simulink model "dft_8_point"  (R2016b)
settings: Solver=VariableStepDiscrete  StartTime=0.0  StopTime=12/fs  RelTol=1e-3  EnableMultiTasking=on
PreLoadFcn:
  | t = 2;
  | b = 14;
  | 
  | fs = 1;
StartFcn:
  | close all;
StopFcn:
  | % create matrices of Re and Im parts over time - inputs
  | xin_re = [xin_0_re xin_1_re xin_2_re xin_3_re xin_4_re xin_5_re xin_6_re xin_7_re];
  | xin_im = [xin_0_im xin_0_im xin_0_im xin_0_im xin_0_im xin_0_im xin_0_im xin_0_im];
  | 
  | % create matrices of Re and Im parts over time - outputs
  | X_re = [X0_re X1_re X2_re X3_re X4_re X5_re X6_re X7_re];
  | X_im = [X0_im X1_im X2_im X3_im X4_im X5_im X6_im X7_im];
  | 
  | % create vectors of Magnitudes and Angles over time
  | X_mag = [X0_mag X1_mag X2_mag X3_mag X4_mag X5_mag X6_mag X7_mag];
  | X_ang = [X0_ang X1_ang X2_ang X3_ang X4_ang X5_ang X6_ang X7_ang];
  | 
  | 
  | figure(1)
  | hold off
  | plot([0:1:7],xin_re(end,:),'r-o','MarkerFaceColor','r');
  | hold on
  | plot([0:1:7],xin_im(end,:),'b-o','MarkerFaceColor','b');
  | xlabel('Samples');
  | ylabel('Magnitude');
  | title('Input to DFT');
  | legend('Real','Imaginary','Location','EastOutside')
  | grid on;
  | 
  | set(1,'Name','Input to DFT','NumberTitle','off');
  | % setStandardFigSize(1);
  | 
  | figure(2)
  | hold off
  | plot([0:1:7],X_mag(end,:),'k-o','MarkerFaceColor','b');
  | hold on
  | xlabel('Frequency Bin');
  | ylabel('Magnitude');
  | grid on;
  | title('Magnitude DFT Plot');
  | 
  | set(2,'Name','Output of DFT','NumberTitle','off');
  | % setStandardFigSize(2);
libraries: xbsIndex_r4 x955
(part 5 of 8)

== system dft_8_point/cplx mult40 ==
  x : Inport
  AddSub : xbsIndex_r4/AddSub  mode=Addition  use_carryin=off  use_carryout=off  en=off  latency=0  precision=User Defined  arith_type="Signed  (2's comp)"  n_bits=t+b+1  bin_pt=b  quantization=Truncate  overflow=Wrap  use_behavioral_HDL=off  hw_selection=Fabric  pipelined=off  dbl_ovrd=off  block_type=addsub
  AddSub1 : xbsIndex_r4/AddSub  mode=Subtraction  use_carryin=off  use_carryout=off  en=off  latency=0  precision=User Defined  arith_type="Signed  (2's comp)"  n_bits=t+b+1  bin_pt=b  quantization=Truncate  overflow=Wrap  use_behavioral_HDL=off  hw_selection=Fabric  pipelined=off  dbl_ovrd=off  block_type=addsub
  Mult{,1..3} (4 alike) : xbsIndex_r4/Mult  precision=User Defined  arith_type="Signed  (2's comp)"  n_bits=t+b  bin_pt=b  quantization=Truncate  overflow=Wrap  en=off  latency=0  use_behavioral_HDL=off  opt=Speed  use_embedded=on  optimum_pipeline=off  pipeline=on  dbl_ovrd=off  use_rpm=on  placement_style=Triangular  block_type=mult
  Reinterpret : xbsIndex_r4/Reinterpret  force_arith_type=on  arith_type="Signed  (2's comp)"  force_bin_pt=on  bin_pt=b  block_type=reinterpret
      settings: infoedit="Changes signal type without altering the binary representation.   You can changed the signal between signed and unsigned, and relocate the binary point.<br><br>Hardware notes: In hardware this block costs nothing.<br><br>Example:  Suppose the input is 6 bits wide, signed, with 2 fractional bits, and the output is forced to unsigned with 0 fractional bits.  Then an input of -2.0 (1110.00 in binary 2's complement) becomes an output of 56 (111000 in binary)."
  Reinterpret1 : xbsIndex_r4/Reinterpret  force_arith_type=on  arith_type="Signed  (2's comp)"  force_bin_pt=on  bin_pt=b  block_type=reinterpret
      settings: infoedit="Changes signal type without altering the binary representation.   You can changed the signal between signed and unsigned, and relocate the binary point.<br><br>Hardware notes: In hardware this block costs nothing.<br><br>Example:  Suppose the input is 6 bits wide, signed, with 2 fractional bits, and the output is forced to unsigned with 0 fractional bits.  Then an input of -2.0 (1110.00 in binary 2's complement) becomes an output of 56 (111000 in binary)."
  W_imaginary : xbsIndex_r4/Constant  const=imag(Wnk)  gui_display_data_type=Fixed-point  arith_type=Signed (2's comp)  n_bits=t+b  bin_pt=b  preci_type=Single  exp_width=8  frac_width=24  explicit_period=off  period=1  equ=P=C  opselect=C  inp2=PCIN>>17  opr=+  inp1=P  carry=CIN  dbl_ovrd=off  block_type=constant
  W_real : xbsIndex_r4/Constant  const=real(Wnk)  gui_display_data_type=Fixed-point  arith_type=Signed (2's comp)  n_bits=t+b  bin_pt=b  preci_type=Single  exp_width=8  frac_width=24  explicit_period=off  period=1  equ=P=C  opselect=C  inp2=PCIN>>17  opr=+  inp1=P  carry=CIN  dbl_ovrd=off  block_type=constant
  x_imaginary : xbsIndex_r4/Slice  nbits=t+b  boolean_output=off  mode=Lower Bit Location + Width  bit1=0  base1=MSB of Input  bit0=0  base0=LSB of Input  dbl_ovrd=off  block_type=slice
  x_real : xbsIndex_r4/Slice  nbits=t+b  boolean_output=off  mode=Upper Bit Location + Width  bit1=0  base1=MSB of Input  bit0=0  base0=LSB of Input  dbl_ovrd=off  block_type=slice
  xWr : Outport
  xWi : Outport  Port=2
  wires:
  x_real/1 -> Reinterpret/1
  x_imaginary/1 -> Reinterpret1/1
  W_real/1 -> Mult1/2, Mult2/2
  x/1 -> x_real/1, x_imaginary/1
  Reinterpret/1 -> Mult/1, Mult2/1
  Reinterpret1/1 -> Mult1/1, Mult3/1
  W_imaginary/1 -> Mult/2, Mult3/2
  AddSub/1 -> xWi/1
  AddSub1/1 -> xWr/1
  Mult/1 -> AddSub/1
  Mult1/1 -> AddSub/2
  Mult3/1 -> AddSub1/2
  Mult2/1 -> AddSub1/1

== system dft_8_point/cplx mult41 ==
  x : Inport
  AddSub : xbsIndex_r4/AddSub  mode=Addition  use_carryin=off  use_carryout=off  en=off  latency=0  precision=User Defined  arith_type="Signed  (2's comp)"  n_bits=t+b+1  bin_pt=b  quantization=Truncate  overflow=Wrap  use_behavioral_HDL=off  hw_selection=Fabric  pipelined=off  dbl_ovrd=off  block_type=addsub
  AddSub1 : xbsIndex_r4/AddSub  mode=Subtraction  use_carryin=off  use_carryout=off  en=off  latency=0  precision=User Defined  arith_type="Signed  (2's comp)"  n_bits=t+b+1  bin_pt=b  quantization=Truncate  overflow=Wrap  use_behavioral_HDL=off  hw_selection=Fabric  pipelined=off  dbl_ovrd=off  block_type=addsub
  Mult{,1..3} (4 alike) : xbsIndex_r4/Mult  precision=User Defined  arith_type="Signed  (2's comp)"  n_bits=t+b  bin_pt=b  quantization=Truncate  overflow=Wrap  en=off  latency=0  use_behavioral_HDL=off  opt=Speed  use_embedded=on  optimum_pipeline=off  pipeline=on  dbl_ovrd=off  use_rpm=on  placement_style=Triangular  block_type=mult
  Reinterpret : xbsIndex_r4/Reinterpret  force_arith_type=on  arith_type="Signed  (2's comp)"  force_bin_pt=on  bin_pt=b  block_type=reinterpret
      settings: infoedit="Changes signal type without altering the binary representation.   You can changed the signal between signed and unsigned, and relocate the binary point.<br><br>Hardware notes: In hardware this block costs nothing.<br><br>Example:  Suppose the input is 6 bits wide, signed, with 2 fractional bits, and the output is forced to unsigned with 0 fractional bits.  Then an input of -2.0 (1110.00 in binary 2's complement) becomes an output of 56 (111000 in binary)."
  Reinterpret1 : xbsIndex_r4/Reinterpret  force_arith_type=on  arith_type="Signed  (2's comp)"  force_bin_pt=on  bin_pt=b  block_type=reinterpret
      settings: infoedit="Changes signal type without altering the binary representation.   You can changed the signal between signed and unsigned, and relocate the binary point.<br><br>Hardware notes: In hardware this block costs nothing.<br><br>Example:  Suppose the input is 6 bits wide, signed, with 2 fractional bits, and the output is forced to unsigned with 0 fractional bits.  Then an input of -2.0 (1110.00 in binary 2's complement) becomes an output of 56 (111000 in binary)."
  W_imaginary : xbsIndex_r4/Constant  const=imag(Wnk)  gui_display_data_type=Fixed-point  arith_type=Signed (2's comp)  n_bits=t+b  bin_pt=b  preci_type=Single  exp_width=8  frac_width=24  explicit_period=off  period=1  equ=P=C  opselect=C  inp2=PCIN>>17  opr=+  inp1=P  carry=CIN  dbl_ovrd=off  block_type=constant
  W_real : xbsIndex_r4/Constant  const=real(Wnk)  gui_display_data_type=Fixed-point  arith_type=Signed (2's comp)  n_bits=t+b  bin_pt=b  preci_type=Single  exp_width=8  frac_width=24  explicit_period=off  period=1  equ=P=C  opselect=C  inp2=PCIN>>17  opr=+  inp1=P  carry=CIN  dbl_ovrd=off  block_type=constant
  x_imaginary : xbsIndex_r4/Slice  nbits=t+b  boolean_output=off  mode=Lower Bit Location + Width  bit1=0  base1=MSB of Input  bit0=0  base0=LSB of Input  dbl_ovrd=off  block_type=slice
  x_real : xbsIndex_r4/Slice  nbits=t+b  boolean_output=off  mode=Upper Bit Location + Width  bit1=0  base1=MSB of Input  bit0=0  base0=LSB of Input  dbl_ovrd=off  block_type=slice
  xWr : Outport
  xWi : Outport  Port=2
  wires:
  x_real/1 -> Reinterpret/1
  x_imaginary/1 -> Reinterpret1/1
  W_real/1 -> Mult1/2, Mult2/2
  x/1 -> x_real/1, x_imaginary/1
  Reinterpret/1 -> Mult/1, Mult2/1
  Reinterpret1/1 -> Mult1/1, Mult3/1
  W_imaginary/1 -> Mult/2, Mult3/2
  AddSub/1 -> xWi/1
  AddSub1/1 -> xWr/1
  Mult/1 -> AddSub/1
  Mult1/1 -> AddSub/2
  Mult3/1 -> AddSub1/2
  Mult2/1 -> AddSub1/1

== system dft_8_point/cplx mult42 ==
  x : Inport
  AddSub : xbsIndex_r4/AddSub  mode=Addition  use_carryin=off  use_carryout=off  en=off  latency=0  precision=User Defined  arith_type="Signed  (2's comp)"  n_bits=t+b+1  bin_pt=b  quantization=Truncate  overflow=Wrap  use_behavioral_HDL=off  hw_selection=Fabric  pipelined=off  dbl_ovrd=off  block_type=addsub
  AddSub1 : xbsIndex_r4/AddSub  mode=Subtraction  use_carryin=off  use_carryout=off  en=off  latency=0  precision=User Defined  arith_type="Signed  (2's comp)"  n_bits=t+b+1  bin_pt=b  quantization=Truncate  overflow=Wrap  use_behavioral_HDL=off  hw_selection=Fabric  pipelined=off  dbl_ovrd=off  block_type=addsub
  Mult{,1..3} (4 alike) : xbsIndex_r4/Mult  precision=User Defined  arith_type="Signed  (2's comp)"  n_bits=t+b  bin_pt=b  quantization=Truncate  overflow=Wrap  en=off  latency=0  use_behavioral_HDL=off  opt=Speed  use_embedded=on  optimum_pipeline=off  pipeline=on  dbl_ovrd=off  use_rpm=on  placement_style=Triangular  block_type=mult
  Reinterpret : xbsIndex_r4/Reinterpret  force_arith_type=on  arith_type="Signed  (2's comp)"  force_bin_pt=on  bin_pt=b  block_type=reinterpret
      settings: infoedit="Changes signal type without altering the binary representation.   You can changed the signal between signed and unsigned, and relocate the binary point.<br><br>Hardware notes: In hardware this block costs nothing.<br><br>Example:  Suppose the input is 6 bits wide, signed, with 2 fractional bits, and the output is forced to unsigned with 0 fractional bits.  Then an input of -2.0 (1110.00 in binary 2's complement) becomes an output of 56 (111000 in binary)."
  Reinterpret1 : xbsIndex_r4/Reinterpret  force_arith_type=on  arith_type="Signed  (2's comp)"  force_bin_pt=on  bin_pt=b  block_type=reinterpret
      settings: infoedit="Changes signal type without altering the binary representation.   You can changed the signal between signed and unsigned, and relocate the binary point.<br><br>Hardware notes: In hardware this block costs nothing.<br><br>Example:  Suppose the input is 6 bits wide, signed, with 2 fractional bits, and the output is forced to unsigned with 0 fractional bits.  Then an input of -2.0 (1110.00 in binary 2's complement) becomes an output of 56 (111000 in binary)."
  W_imaginary : xbsIndex_r4/Constant  const=imag(Wnk)  gui_display_data_type=Fixed-point  arith_type=Signed (2's comp)  n_bits=t+b  bin_pt=b  preci_type=Single  exp_width=8  frac_width=24  explicit_period=off  period=1  equ=P=C  opselect=C  inp2=PCIN>>17  opr=+  inp1=P  carry=CIN  dbl_ovrd=off  block_type=constant
  W_real : xbsIndex_r4/Constant  const=real(Wnk)  gui_display_data_type=Fixed-point  arith_type=Signed (2's comp)  n_bits=t+b  bin_pt=b  preci_type=Single  exp_width=8  frac_width=24  explicit_period=off  period=1  equ=P=C  opselect=C  inp2=PCIN>>17  opr=+  inp1=P  carry=CIN  dbl_ovrd=off  block_type=constant
  x_imaginary : xbsIndex_r4/Slice  nbits=t+b  boolean_output=off  mode=Lower Bit Location + Width  bit1=0  base1=MSB of Input  bit0=0  base0=LSB of Input  dbl_ovrd=off  block_type=slice
  x_real : xbsIndex_r4/Slice  nbits=t+b  boolean_output=off  mode=Upper Bit Location + Width  bit1=0  base1=MSB of Input  bit0=0  base0=LSB of Input  dbl_ovrd=off  block_type=slice
  xWr : Outport
  xWi : Outport  Port=2
  wires:
  x_real/1 -> Reinterpret/1
  x_imaginary/1 -> Reinterpret1/1
  W_real/1 -> Mult1/2, Mult2/2
  x/1 -> x_real/1, x_imaginary/1
  Reinterpret/1 -> Mult/1, Mult2/1
  Reinterpret1/1 -> Mult1/1, Mult3/1
  W_imaginary/1 -> Mult/2, Mult3/2
  AddSub/1 -> xWi/1
  AddSub1/1 -> xWr/1
  Mult/1 -> AddSub/1
  Mult1/1 -> AddSub/2
  Mult3/1 -> AddSub1/2
  Mult2/1 -> AddSub1/1

== system dft_8_point/cplx mult43 ==
  x : Inport
  AddSub : xbsIndex_r4/AddSub  mode=Addition  use_carryin=off  use_carryout=off  en=off  latency=0  precision=User Defined  arith_type="Signed  (2's comp)"  n_bits=t+b+1  bin_pt=b  quantization=Truncate  overflow=Wrap  use_behavioral_HDL=off  hw_selection=Fabric  pipelined=off  dbl_ovrd=off  block_type=addsub
  AddSub1 : xbsIndex_r4/AddSub  mode=Subtraction  use_carryin=off  use_carryout=off  en=off  latency=0  precision=User Defined  arith_type="Signed  (2's comp)"  n_bits=t+b+1  bin_pt=b  quantization=Truncate  overflow=Wrap  use_behavioral_HDL=off  hw_selection=Fabric  pipelined=off  dbl_ovrd=off  block_type=addsub
  Mult{,1..3} (4 alike) : xbsIndex_r4/Mult  precision=User Defined  arith_type="Signed  (2's comp)"  n_bits=t+b  bin_pt=b  quantization=Truncate  overflow=Wrap  en=off  latency=0  use_behavioral_HDL=off  opt=Speed  use_embedded=on  optimum_pipeline=off  pipeline=on  dbl_ovrd=off  use_rpm=on  placement_style=Triangular  block_type=mult
  Reinterpret : xbsIndex_r4/Reinterpret  force_arith_type=on  arith_type="Signed  (2's comp)"  force_bin_pt=on  bin_pt=b  block_type=reinterpret
      settings: infoedit="Changes signal type without altering the binary representation.   You can changed the signal between signed and unsigned, and relocate the binary point.<br><br>Hardware notes: In hardware this block costs nothing.<br><br>Example:  Suppose the input is 6 bits wide, signed, with 2 fractional bits, and the output is forced to unsigned with 0 fractional bits.  Then an input of -2.0 (1110.00 in binary 2's complement) becomes an output of 56 (111000 in binary)."
  Reinterpret1 : xbsIndex_r4/Reinterpret  force_arith_type=on  arith_type="Signed  (2's comp)"  force_bin_pt=on  bin_pt=b  block_type=reinterpret
      settings: infoedit="Changes signal type without altering the binary representation.   You can changed the signal between signed and unsigned, and relocate the binary point.<br><br>Hardware notes: In hardware this block costs nothing.<br><br>Example:  Suppose the input is 6 bits wide, signed, with 2 fractional bits, and the output is forced to unsigned with 0 fractional bits.  Then an input of -2.0 (1110.00 in binary 2's complement) becomes an output of 56 (111000 in binary)."
  W_imaginary : xbsIndex_r4/Constant  const=imag(Wnk)  gui_display_data_type=Fixed-point  arith_type=Signed (2's comp)  n_bits=t+b  bin_pt=b  preci_type=Single  exp_width=8  frac_width=24  explicit_period=off  period=1  equ=P=C  opselect=C  inp2=PCIN>>17  opr=+  inp1=P  carry=CIN  dbl_ovrd=off  block_type=constant
  W_real : xbsIndex_r4/Constant  const=real(Wnk)  gui_display_data_type=Fixed-point  arith_type=Signed (2's comp)  n_bits=t+b  bin_pt=b  preci_type=Single  exp_width=8  frac_width=24  explicit_period=off  period=1  equ=P=C  opselect=C  inp2=PCIN>>17  opr=+  inp1=P  carry=CIN  dbl_ovrd=off  block_type=constant
  x_imaginary : xbsIndex_r4/Slice  nbits=t+b  boolean_output=off  mode=Lower Bit Location + Width  bit1=0  base1=MSB of Input  bit0=0  base0=LSB of Input  dbl_ovrd=off  block_type=slice
  x_real : xbsIndex_r4/Slice  nbits=t+b  boolean_output=off  mode=Upper Bit Location + Width  bit1=0  base1=MSB of Input  bit0=0  base0=LSB of Input  dbl_ovrd=off  block_type=slice
  xWr : Outport
  xWi : Outport  Port=2
  wires:
  x_real/1 -> Reinterpret/1
  x_imaginary/1 -> Reinterpret1/1
  W_real/1 -> Mult1/2, Mult2/2
  x/1 -> x_real/1, x_imaginary/1
  Reinterpret/1 -> Mult/1, Mult2/1
  Reinterpret1/1 -> Mult1/1, Mult3/1
  W_imaginary/1 -> Mult/2, Mult3/2
  AddSub/1 -> xWi/1
  AddSub1/1 -> xWr/1
  Mult/1 -> AddSub/1
  Mult1/1 -> AddSub/2
  Mult3/1 -> AddSub1/2
  Mult2/1 -> AddSub1/1

== system dft_8_point/cplx mult44 ==
  x : Inport
  AddSub : xbsIndex_r4/AddSub  mode=Addition  use_carryin=off  use_carryout=off  en=off  latency=0  precision=User Defined  arith_type="Signed  (2's comp)"  n_bits=t+b+1  bin_pt=b  quantization=Truncate  overflow=Wrap  use_behavioral_HDL=off  hw_selection=Fabric  pipelined=off  dbl_ovrd=off  block_type=addsub
  AddSub1 : xbsIndex_r4/AddSub  mode=Subtraction  use_carryin=off  use_carryout=off  en=off  latency=0  precision=User Defined  arith_type="Signed  (2's comp)"  n_bits=t+b+1  bin_pt=b  quantization=Truncate  overflow=Wrap  use_behavioral_HDL=off  hw_selection=Fabric  pipelined=off  dbl_ovrd=off  block_type=addsub
  Mult{,1..3} (4 alike) : xbsIndex_r4/Mult  precision=User Defined  arith_type="Signed  (2's comp)"  n_bits=t+b  bin_pt=b  quantization=Truncate  overflow=Wrap  en=off  latency=0  use_behavioral_HDL=off  opt=Speed  use_embedded=on  optimum_pipeline=off  pipeline=on  dbl_ovrd=off  use_rpm=on  placement_style=Triangular  block_type=mult
  Reinterpret : xbsIndex_r4/Reinterpret  force_arith_type=on  arith_type="Signed  (2's comp)"  force_bin_pt=on  bin_pt=b  block_type=reinterpret
      settings: infoedit="Changes signal type without altering the binary representation.   You can changed the signal between signed and unsigned, and relocate the binary point.<br><br>Hardware notes: In hardware this block costs nothing.<br><br>Example:  Suppose the input is 6 bits wide, signed, with 2 fractional bits, and the output is forced to unsigned with 0 fractional bits.  Then an input of -2.0 (1110.00 in binary 2's complement) becomes an output of 56 (111000 in binary)."
  Reinterpret1 : xbsIndex_r4/Reinterpret  force_arith_type=on  arith_type="Signed  (2's comp)"  force_bin_pt=on  bin_pt=b  block_type=reinterpret
      settings: infoedit="Changes signal type without altering the binary representation.   You can changed the signal between signed and unsigned, and relocate the binary point.<br><br>Hardware notes: In hardware this block costs nothing.<br><br>Example:  Suppose the input is 6 bits wide, signed, with 2 fractional bits, and the output is forced to unsigned with 0 fractional bits.  Then an input of -2.0 (1110.00 in binary 2's complement) becomes an output of 56 (111000 in binary)."
  W_imaginary : xbsIndex_r4/Constant  const=imag(Wnk)  gui_display_data_type=Fixed-point  arith_type=Signed (2's comp)  n_bits=t+b  bin_pt=b  preci_type=Single  exp_width=8  frac_width=24  explicit_period=off  period=1  equ=P=C  opselect=C  inp2=PCIN>>17  opr=+  inp1=P  carry=CIN  dbl_ovrd=off  block_type=constant
  W_real : xbsIndex_r4/Constant  const=real(Wnk)  gui_display_data_type=Fixed-point  arith_type=Signed (2's comp)  n_bits=t+b  bin_pt=b  preci_type=Single  exp_width=8  frac_width=24  explicit_period=off  period=1  equ=P=C  opselect=C  inp2=PCIN>>17  opr=+  inp1=P  carry=CIN  dbl_ovrd=off  block_type=constant
  x_imaginary : xbsIndex_r4/Slice  nbits=t+b  boolean_output=off  mode=Lower Bit Location + Width  bit1=0  base1=MSB of Input  bit0=0  base0=LSB of Input  dbl_ovrd=off  block_type=slice
  x_real : xbsIndex_r4/Slice  nbits=t+b  boolean_output=off  mode=Upper Bit Location + Width  bit1=0  base1=MSB of Input  bit0=0  base0=LSB of Input  dbl_ovrd=off  block_type=slice
  xWr : Outport
  xWi : Outport  Port=2
  wires:
  x_real/1 -> Reinterpret/1
  x_imaginary/1 -> Reinterpret1/1
  W_real/1 -> Mult1/2, Mult2/2
  x/1 -> x_real/1, x_imaginary/1
  Reinterpret/1 -> Mult/1, Mult2/1
  Reinterpret1/1 -> Mult1/1, Mult3/1
  W_imaginary/1 -> Mult/2, Mult3/2
  AddSub/1 -> xWi/1
  AddSub1/1 -> xWr/1
  Mult/1 -> AddSub/1
  Mult1/1 -> AddSub/2
  Mult3/1 -> AddSub1/2
  Mult2/1 -> AddSub1/1

== system dft_8_point/cplx mult45 ==
  x : Inport
  AddSub : xbsIndex_r4/AddSub  mode=Addition  use_carryin=off  use_carryout=off  en=off  latency=0  precision=User Defined  arith_type="Signed  (2's comp)"  n_bits=t+b+1  bin_pt=b  quantization=Truncate  overflow=Wrap  use_behavioral_HDL=off  hw_selection=Fabric  pipelined=off  dbl_ovrd=off  block_type=addsub
  AddSub1 : xbsIndex_r4/AddSub  mode=Subtraction  use_carryin=off  use_carryout=off  en=off  latency=0  precision=User Defined  arith_type="Signed  (2's comp)"  n_bits=t+b+1  bin_pt=b  quantization=Truncate  overflow=Wrap  use_behavioral_HDL=off  hw_selection=Fabric  pipelined=off  dbl_ovrd=off  block_type=addsub
  Mult{,1..3} (4 alike) : xbsIndex_r4/Mult  precision=User Defined  arith_type="Signed  (2's comp)"  n_bits=t+b  bin_pt=b  quantization=Truncate  overflow=Wrap  en=off  latency=0  use_behavioral_HDL=off  opt=Speed  use_embedded=on  optimum_pipeline=off  pipeline=on  dbl_ovrd=off  use_rpm=on  placement_style=Triangular  block_type=mult
  Reinterpret : xbsIndex_r4/Reinterpret  force_arith_type=on  arith_type="Signed  (2's comp)"  force_bin_pt=on  bin_pt=b  block_type=reinterpret
      settings: infoedit="Changes signal type without altering the binary representation.   You can changed the signal between signed and unsigned, and relocate the binary point.<br><br>Hardware notes: In hardware this block costs nothing.<br><br>Example:  Suppose the input is 6 bits wide, signed, with 2 fractional bits, and the output is forced to unsigned with 0 fractional bits.  Then an input of -2.0 (1110.00 in binary 2's complement) becomes an output of 56 (111000 in binary)."
  Reinterpret1 : xbsIndex_r4/Reinterpret  force_arith_type=on  arith_type="Signed  (2's comp)"  force_bin_pt=on  bin_pt=b  block_type=reinterpret
      settings: infoedit="Changes signal type without altering the binary representation.   You can changed the signal between signed and unsigned, and relocate the binary point.<br><br>Hardware notes: In hardware this block costs nothing.<br><br>Example:  Suppose the input is 6 bits wide, signed, with 2 fractional bits, and the output is forced to unsigned with 0 fractional bits.  Then an input of -2.0 (1110.00 in binary 2's complement) becomes an output of 56 (111000 in binary)."
  W_imaginary : xbsIndex_r4/Constant  const=imag(Wnk)  gui_display_data_type=Fixed-point  arith_type=Signed (2's comp)  n_bits=t+b  bin_pt=b  preci_type=Single  exp_width=8  frac_width=24  explicit_period=off  period=1  equ=P=C  opselect=C  inp2=PCIN>>17  opr=+  inp1=P  carry=CIN  dbl_ovrd=off  block_type=constant
  W_real : xbsIndex_r4/Constant  const=real(Wnk)  gui_display_data_type=Fixed-point  arith_type=Signed (2's comp)  n_bits=t+b  bin_pt=b  preci_type=Single  exp_width=8  frac_width=24  explicit_period=off  period=1  equ=P=C  opselect=C  inp2=PCIN>>17  opr=+  inp1=P  carry=CIN  dbl_ovrd=off  block_type=constant
  x_imaginary : xbsIndex_r4/Slice  nbits=t+b  boolean_output=off  mode=Lower Bit Location + Width  bit1=0  base1=MSB of Input  bit0=0  base0=LSB of Input  dbl_ovrd=off  block_type=slice
  x_real : xbsIndex_r4/Slice  nbits=t+b  boolean_output=off  mode=Upper Bit Location + Width  bit1=0  base1=MSB of Input  bit0=0  base0=LSB of Input  dbl_ovrd=off  block_type=slice
  xWr : Outport
  xWi : Outport  Port=2
  wires:
  x_real/1 -> Reinterpret/1
  x_imaginary/1 -> Reinterpret1/1
  W_real/1 -> Mult1/2, Mult2/2
  x/1 -> x_real/1, x_imaginary/1
  Reinterpret/1 -> Mult/1, Mult2/1
  Reinterpret1/1 -> Mult1/1, Mult3/1
  W_imaginary/1 -> Mult/2, Mult3/2
  AddSub/1 -> xWi/1
  AddSub1/1 -> xWr/1
  Mult/1 -> AddSub/1
  Mult1/1 -> AddSub/2
  Mult3/1 -> AddSub1/2
  Mult2/1 -> AddSub1/1

== system dft_8_point/cplx mult46 ==
  x : Inport
  AddSub : xbsIndex_r4/AddSub  mode=Addition  use_carryin=off  use_carryout=off  en=off  latency=0  precision=User Defined  arith_type="Signed  (2's comp)"  n_bits=t+b+1  bin_pt=b  quantization=Truncate  overflow=Wrap  use_behavioral_HDL=off  hw_selection=Fabric  pipelined=off  dbl_ovrd=off  block_type=addsub
  AddSub1 : xbsIndex_r4/AddSub  mode=Subtraction  use_carryin=off  use_carryout=off  en=off  latency=0  precision=User Defined  arith_type="Signed  (2's comp)"  n_bits=t+b+1  bin_pt=b  quantization=Truncate  overflow=Wrap  use_behavioral_HDL=off  hw_selection=Fabric  pipelined=off  dbl_ovrd=off  block_type=addsub
  Mult{,1..3} (4 alike) : xbsIndex_r4/Mult  precision=User Defined  arith_type="Signed  (2's comp)"  n_bits=t+b  bin_pt=b  quantization=Truncate  overflow=Wrap  en=off  latency=0  use_behavioral_HDL=off  opt=Speed  use_embedded=on  optimum_pipeline=off  pipeline=on  dbl_ovrd=off  use_rpm=on  placement_style=Triangular  block_type=mult
  Reinterpret : xbsIndex_r4/Reinterpret  force_arith_type=on  arith_type="Signed  (2's comp)"  force_bin_pt=on  bin_pt=b  block_type=reinterpret
      settings: infoedit="Changes signal type without altering the binary representation.   You can changed the signal between signed and unsigned, and relocate the binary point.<br><br>Hardware notes: In hardware this block costs nothing.<br><br>Example:  Suppose the input is 6 bits wide, signed, with 2 fractional bits, and the output is forced to unsigned with 0 fractional bits.  Then an input of -2.0 (1110.00 in binary 2's complement) becomes an output of 56 (111000 in binary)."
  Reinterpret1 : xbsIndex_r4/Reinterpret  force_arith_type=on  arith_type="Signed  (2's comp)"  force_bin_pt=on  bin_pt=b  block_type=reinterpret
      settings: infoedit="Changes signal type without altering the binary representation.   You can changed the signal between signed and unsigned, and relocate the binary point.<br><br>Hardware notes: In hardware this block costs nothing.<br><br>Example:  Suppose the input is 6 bits wide, signed, with 2 fractional bits, and the output is forced to unsigned with 0 fractional bits.  Then an input of -2.0 (1110.00 in binary 2's complement) becomes an output of 56 (111000 in binary)."
  W_imaginary : xbsIndex_r4/Constant  const=imag(Wnk)  gui_display_data_type=Fixed-point  arith_type=Signed (2's comp)  n_bits=t+b  bin_pt=b  preci_type=Single  exp_width=8  frac_width=24  explicit_period=off  period=1  equ=P=C  opselect=C  inp2=PCIN>>17  opr=+  inp1=P  carry=CIN  dbl_ovrd=off  block_type=constant
  W_real : xbsIndex_r4/Constant  const=real(Wnk)  gui_display_data_type=Fixed-point  arith_type=Signed (2's comp)  n_bits=t+b  bin_pt=b  preci_type=Single  exp_width=8  frac_width=24  explicit_period=off  period=1  equ=P=C  opselect=C  inp2=PCIN>>17  opr=+  inp1=P  carry=CIN  dbl_ovrd=off  block_type=constant
  x_imaginary : xbsIndex_r4/Slice  nbits=t+b  boolean_output=off  mode=Lower Bit Location + Width  bit1=0  base1=MSB of Input  bit0=0  base0=LSB of Input  dbl_ovrd=off  block_type=slice
  x_real : xbsIndex_r4/Slice  nbits=t+b  boolean_output=off  mode=Upper Bit Location + Width  bit1=0  base1=MSB of Input  bit0=0  base0=LSB of Input  dbl_ovrd=off  block_type=slice
  xWr : Outport
  xWi : Outport  Port=2
  wires:
  x_real/1 -> Reinterpret/1
  x_imaginary/1 -> Reinterpret1/1
  W_real/1 -> Mult1/2, Mult2/2
  x/1 -> x_real/1, x_imaginary/1
  Reinterpret/1 -> Mult/1, Mult2/1
  Reinterpret1/1 -> Mult1/1, Mult3/1
  W_imaginary/1 -> Mult/2, Mult3/2
  AddSub/1 -> xWi/1
  AddSub1/1 -> xWr/1
  Mult/1 -> AddSub/1
  Mult1/1 -> AddSub/2
  Mult3/1 -> AddSub1/2
  Mult2/1 -> AddSub1/1

== system dft_8_point/cplx mult47 ==
  x : Inport
  AddSub : xbsIndex_r4/AddSub  mode=Addition  use_carryin=off  use_carryout=off  en=off  latency=0  precision=User Defined  arith_type="Signed  (2's comp)"  n_bits=t+b+1  bin_pt=b  quantization=Truncate  overflow=Wrap  use_behavioral_HDL=off  hw_selection=Fabric  pipelined=off  dbl_ovrd=off  block_type=addsub
  AddSub1 : xbsIndex_r4/AddSub  mode=Subtraction  use_carryin=off  use_carryout=off  en=off  latency=0  precision=User Defined  arith_type="Signed  (2's comp)"  n_bits=t+b+1  bin_pt=b  quantization=Truncate  overflow=Wrap  use_behavioral_HDL=off  hw_selection=Fabric  pipelined=off  dbl_ovrd=off  block_type=addsub
  Mult{,1..3} (4 alike) : xbsIndex_r4/Mult  precision=User Defined  arith_type="Signed  (2's comp)"  n_bits=t+b  bin_pt=b  quantization=Truncate  overflow=Wrap  en=off  latency=0  use_behavioral_HDL=off  opt=Speed  use_embedded=on  optimum_pipeline=off  pipeline=on  dbl_ovrd=off  use_rpm=on  placement_style=Triangular  block_type=mult
  Reinterpret : xbsIndex_r4/Reinterpret  force_arith_type=on  arith_type="Signed  (2's comp)"  force_bin_pt=on  bin_pt=b  block_type=reinterpret
      settings: infoedit="Changes signal type without altering the binary representation.   You can changed the signal between signed and unsigned, and relocate the binary point.<br><br>Hardware notes: In hardware this block costs nothing.<br><br>Example:  Suppose the input is 6 bits wide, signed, with 2 fractional bits, and the output is forced to unsigned with 0 fractional bits.  Then an input of -2.0 (1110.00 in binary 2's complement) becomes an output of 56 (111000 in binary)."
  Reinterpret1 : xbsIndex_r4/Reinterpret  force_arith_type=on  arith_type="Signed  (2's comp)"  force_bin_pt=on  bin_pt=b  block_type=reinterpret
      settings: infoedit="Changes signal type without altering the binary representation.   You can changed the signal between signed and unsigned, and relocate the binary point.<br><br>Hardware notes: In hardware this block costs nothing.<br><br>Example:  Suppose the input is 6 bits wide, signed, with 2 fractional bits, and the output is forced to unsigned with 0 fractional bits.  Then an input of -2.0 (1110.00 in binary 2's complement) becomes an output of 56 (111000 in binary)."
  W_imaginary : xbsIndex_r4/Constant  const=imag(Wnk)  gui_display_data_type=Fixed-point  arith_type=Signed (2's comp)  n_bits=t+b  bin_pt=b  preci_type=Single  exp_width=8  frac_width=24  explicit_period=off  period=1  equ=P=C  opselect=C  inp2=PCIN>>17  opr=+  inp1=P  carry=CIN  dbl_ovrd=off  block_type=constant
  W_real : xbsIndex_r4/Constant  const=real(Wnk)  gui_display_data_type=Fixed-point  arith_type=Signed (2's comp)  n_bits=t+b  bin_pt=b  preci_type=Single  exp_width=8  frac_width=24  explicit_period=off  period=1  equ=P=C  opselect=C  inp2=PCIN>>17  opr=+  inp1=P  carry=CIN  dbl_ovrd=off  block_type=constant
  x_imaginary : xbsIndex_r4/Slice  nbits=t+b  boolean_output=off  mode=Lower Bit Location + Width  bit1=0  base1=MSB of Input  bit0=0  base0=LSB of Input  dbl_ovrd=off  block_type=slice
  x_real : xbsIndex_r4/Slice  nbits=t+b  boolean_output=off  mode=Upper Bit Location + Width  bit1=0  base1=MSB of Input  bit0=0  base0=LSB of Input  dbl_ovrd=off  block_type=slice
  xWr : Outport
  xWi : Outport  Port=2
  wires:
  x_real/1 -> Reinterpret/1
  x_imaginary/1 -> Reinterpret1/1
  W_real/1 -> Mult1/2, Mult2/2
  x/1 -> x_real/1, x_imaginary/1
  Reinterpret/1 -> Mult/1, Mult2/1
  Reinterpret1/1 -> Mult1/1, Mult3/1
  W_imaginary/1 -> Mult/2, Mult3/2
  AddSub/1 -> xWi/1
  AddSub1/1 -> xWr/1
  Mult/1 -> AddSub/1
  Mult1/1 -> AddSub/2
  Mult3/1 -> AddSub1/2
  Mult2/1 -> AddSub1/1

== system dft_8_point/cplx mult48 ==
  x : Inport
  AddSub : xbsIndex_r4/AddSub  mode=Addition  use_carryin=off  use_carryout=off  en=off  latency=0  precision=User Defined  arith_type="Signed  (2's comp)"  n_bits=t+b+1  bin_pt=b  quantization=Truncate  overflow=Wrap  use_behavioral_HDL=off  hw_selection=Fabric  pipelined=off  dbl_ovrd=off  block_type=addsub
  AddSub1 : xbsIndex_r4/AddSub  mode=Subtraction  use_carryin=off  use_carryout=off  en=off  latency=0  precision=User Defined  arith_type="Signed  (2's comp)"  n_bits=t+b+1  bin_pt=b  quantization=Truncate  overflow=Wrap  use_behavioral_HDL=off  hw_selection=Fabric  pipelined=off  dbl_ovrd=off  block_type=addsub
  Mult{,1..3} (4 alike) : xbsIndex_r4/Mult  precision=User Defined  arith_type="Signed  (2's comp)"  n_bits=t+b  bin_pt=b  quantization=Truncate  overflow=Wrap  en=off  latency=0  use_behavioral_HDL=off  opt=Speed  use_embedded=on  optimum_pipeline=off  pipeline=on  dbl_ovrd=off  use_rpm=on  placement_style=Triangular  block_type=mult
  Reinterpret : xbsIndex_r4/Reinterpret  force_arith_type=on  arith_type="Signed  (2's comp)"  force_bin_pt=on  bin_pt=b  block_type=reinterpret
      settings: infoedit="Changes signal type without altering the binary representation.   You can changed the signal between signed and unsigned, and relocate the binary point.<br><br>Hardware notes: In hardware this block costs nothing.<br><br>Example:  Suppose the input is 6 bits wide, signed, with 2 fractional bits, and the output is forced to unsigned with 0 fractional bits.  Then an input of -2.0 (1110.00 in binary 2's complement) becomes an output of 56 (111000 in binary)."
  Reinterpret1 : xbsIndex_r4/Reinterpret  force_arith_type=on  arith_type="Signed  (2's comp)"  force_bin_pt=on  bin_pt=b  block_type=reinterpret
      settings: infoedit="Changes signal type without altering the binary representation.   You can changed the signal between signed and unsigned, and relocate the binary point.<br><br>Hardware notes: In hardware this block costs nothing.<br><br>Example:  Suppose the input is 6 bits wide, signed, with 2 fractional bits, and the output is forced to unsigned with 0 fractional bits.  Then an input of -2.0 (1110.00 in binary 2's complement) becomes an output of 56 (111000 in binary)."
  W_imaginary : xbsIndex_r4/Constant  const=imag(Wnk)  gui_display_data_type=Fixed-point  arith_type=Signed (2's comp)  n_bits=t+b  bin_pt=b  preci_type=Single  exp_width=8  frac_width=24  explicit_period=off  period=1  equ=P=C  opselect=C  inp2=PCIN>>17  opr=+  inp1=P  carry=CIN  dbl_ovrd=off  block_type=constant
  W_real : xbsIndex_r4/Constant  const=real(Wnk)  gui_display_data_type=Fixed-point  arith_type=Signed (2's comp)  n_bits=t+b  bin_pt=b  preci_type=Single  exp_width=8  frac_width=24  explicit_period=off  period=1  equ=P=C  opselect=C  inp2=PCIN>>17  opr=+  inp1=P  carry=CIN  dbl_ovrd=off  block_type=constant
  x_imaginary : xbsIndex_r4/Slice  nbits=t+b  boolean_output=off  mode=Lower Bit Location + Width  bit1=0  base1=MSB of Input  bit0=0  base0=LSB of Input  dbl_ovrd=off  block_type=slice
  x_real : xbsIndex_r4/Slice  nbits=t+b  boolean_output=off  mode=Upper Bit Location + Width  bit1=0  base1=MSB of Input  bit0=0  base0=LSB of Input  dbl_ovrd=off  block_type=slice
  xWr : Outport
  xWi : Outport  Port=2
  wires:
  x_real/1 -> Reinterpret/1
  x_imaginary/1 -> Reinterpret1/1
  W_real/1 -> Mult1/2, Mult2/2
  x/1 -> x_real/1, x_imaginary/1
  Reinterpret/1 -> Mult/1, Mult2/1
  Reinterpret1/1 -> Mult1/1, Mult3/1
  W_imaginary/1 -> Mult/2, Mult3/2
  AddSub/1 -> xWi/1
  AddSub1/1 -> xWr/1
  Mult/1 -> AddSub/1
  Mult1/1 -> AddSub/2
  Mult3/1 -> AddSub1/2
  Mult2/1 -> AddSub1/1

== system dft_8_point/cplx mult49 ==
  x : Inport
  AddSub : xbsIndex_r4/AddSub  mode=Addition  use_carryin=off  use_carryout=off  en=off  latency=0  precision=User Defined  arith_type="Signed  (2's comp)"  n_bits=t+b+1  bin_pt=b  quantization=Truncate  overflow=Wrap  use_behavioral_HDL=off  hw_selection=Fabric  pipelined=off  dbl_ovrd=off  block_type=addsub
  AddSub1 : xbsIndex_r4/AddSub  mode=Subtraction  use_carryin=off  use_carryout=off  en=off  latency=0  precision=User Defined  arith_type="Signed  (2's comp)"  n_bits=t+b+1  bin_pt=b  quantization=Truncate  overflow=Wrap  use_behavioral_HDL=off  hw_selection=Fabric  pipelined=off  dbl_ovrd=off  block_type=addsub
  Mult{,1..3} (4 alike) : xbsIndex_r4/Mult  precision=User Defined  arith_type="Signed  (2's comp)"  n_bits=t+b  bin_pt=b  quantization=Truncate  overflow=Wrap  en=off  latency=0  use_behavioral_HDL=off  opt=Speed  use_embedded=on  optimum_pipeline=off  pipeline=on  dbl_ovrd=off  use_rpm=on  placement_style=Triangular  block_type=mult
  Reinterpret : xbsIndex_r4/Reinterpret  force_arith_type=on  arith_type="Signed  (2's comp)"  force_bin_pt=on  bin_pt=b  block_type=reinterpret
      settings: infoedit="Changes signal type without altering the binary representation.   You can changed the signal between signed and unsigned, and relocate the binary point.<br><br>Hardware notes: In hardware this block costs nothing.<br><br>Example:  Suppose the input is 6 bits wide, signed, with 2 fractional bits, and the output is forced to unsigned with 0 fractional bits.  Then an input of -2.0 (1110.00 in binary 2's complement) becomes an output of 56 (111000 in binary)."
  Reinterpret1 : xbsIndex_r4/Reinterpret  force_arith_type=on  arith_type="Signed  (2's comp)"  force_bin_pt=on  bin_pt=b  block_type=reinterpret
      settings: infoedit="Changes signal type without altering the binary representation.   You can changed the signal between signed and unsigned, and relocate the binary point.<br><br>Hardware notes: In hardware this block costs nothing.<br><br>Example:  Suppose the input is 6 bits wide, signed, with 2 fractional bits, and the output is forced to unsigned with 0 fractional bits.  Then an input of -2.0 (1110.00 in binary 2's complement) becomes an output of 56 (111000 in binary)."
  W_imaginary : xbsIndex_r4/Constant  const=imag(Wnk)  gui_display_data_type=Fixed-point  arith_type=Signed (2's comp)  n_bits=t+b  bin_pt=b  preci_type=Single  exp_width=8  frac_width=24  explicit_period=off  period=1  equ=P=C  opselect=C  inp2=PCIN>>17  opr=+  inp1=P  carry=CIN  dbl_ovrd=off  block_type=constant
  W_real : xbsIndex_r4/Constant  const=real(Wnk)  gui_display_data_type=Fixed-point  arith_type=Signed (2's comp)  n_bits=t+b  bin_pt=b  preci_type=Single  exp_width=8  frac_width=24  explicit_period=off  period=1  equ=P=C  opselect=C  inp2=PCIN>>17  opr=+  inp1=P  carry=CIN  dbl_ovrd=off  block_type=constant
  x_imaginary : xbsIndex_r4/Slice  nbits=t+b  boolean_output=off  mode=Lower Bit Location + Width  bit1=0  base1=MSB of Input  bit0=0  base0=LSB of Input  dbl_ovrd=off  block_type=slice
  x_real : xbsIndex_r4/Slice  nbits=t+b  boolean_output=off  mode=Upper Bit Location + Width  bit1=0  base1=MSB of Input  bit0=0  base0=LSB of Input  dbl_ovrd=off  block_type=slice
  xWr : Outport
  xWi : Outport  Port=2
  wires:
  x_real/1 -> Reinterpret/1
  x_imaginary/1 -> Reinterpret1/1
  W_real/1 -> Mult1/2, Mult2/2
  x/1 -> x_real/1, x_imaginary/1
  Reinterpret/1 -> Mult/1, Mult2/1
  Reinterpret1/1 -> Mult1/1, Mult3/1
  W_imaginary/1 -> Mult/2, Mult3/2
  AddSub/1 -> xWi/1
  AddSub1/1 -> xWr/1
  Mult/1 -> AddSub/1
  Mult1/1 -> AddSub/2
  Mult3/1 -> AddSub1/2
  Mult2/1 -> AddSub1/1

== system dft_8_point/cplx mult5 ==
  x : Inport
  AddSub : xbsIndex_r4/AddSub  mode=Addition  use_carryin=off  use_carryout=off  en=off  latency=0  precision=User Defined  arith_type="Signed  (2's comp)"  n_bits=t+b+1  bin_pt=b  quantization=Truncate  overflow=Wrap  use_behavioral_HDL=off  hw_selection=Fabric  pipelined=off  dbl_ovrd=off  block_type=addsub
  AddSub1 : xbsIndex_r4/AddSub  mode=Subtraction  use_carryin=off  use_carryout=off  en=off  latency=0  precision=User Defined  arith_type="Signed  (2's comp)"  n_bits=t+b+1  bin_pt=b  quantization=Truncate  overflow=Wrap  use_behavioral_HDL=off  hw_selection=Fabric  pipelined=off  dbl_ovrd=off  block_type=addsub
  Mult{,1..3} (4 alike) : xbsIndex_r4/Mult  precision=User Defined  arith_type="Signed  (2's comp)"  n_bits=t+b  bin_pt=b  quantization=Truncate  overflow=Wrap  en=off  latency=0  use_behavioral_HDL=off  opt=Speed  use_embedded=on  optimum_pipeline=off  pipeline=on  dbl_ovrd=off  use_rpm=on  placement_style=Triangular  block_type=mult
  Reinterpret : xbsIndex_r4/Reinterpret  force_arith_type=on  arith_type="Signed  (2's comp)"  force_bin_pt=on  bin_pt=b  block_type=reinterpret
      settings: infoedit="Changes signal type without altering the binary representation.   You can changed the signal between signed and unsigned, and relocate the binary point.<br><br>Hardware notes: In hardware this block costs nothing.<br><br>Example:  Suppose the input is 6 bits wide, signed, with 2 fractional bits, and the output is forced to unsigned with 0 fractional bits.  Then an input of -2.0 (1110.00 in binary 2's complement) becomes an output of 56 (111000 in binary)."
  Reinterpret1 : xbsIndex_r4/Reinterpret  force_arith_type=on  arith_type="Signed  (2's comp)"  force_bin_pt=on  bin_pt=b  block_type=reinterpret
      settings: infoedit="Changes signal type without altering the binary representation.   You can changed the signal between signed and unsigned, and relocate the binary point.<br><br>Hardware notes: In hardware this block costs nothing.<br><br>Example:  Suppose the input is 6 bits wide, signed, with 2 fractional bits, and the output is forced to unsigned with 0 fractional bits.  Then an input of -2.0 (1110.00 in binary 2's complement) becomes an output of 56 (111000 in binary)."
  W_imaginary : xbsIndex_r4/Constant  const=imag(Wnk)  gui_display_data_type=Fixed-point  arith_type=Signed (2's comp)  n_bits=t+b  bin_pt=b  preci_type=Single  exp_width=8  frac_width=24  explicit_period=off  period=1  equ=P=C  opselect=C  inp2=PCIN>>17  opr=+  inp1=P  carry=CIN  dbl_ovrd=off  block_type=constant
  W_real : xbsIndex_r4/Constant  const=real(Wnk)  gui_display_data_type=Fixed-point  arith_type=Signed (2's comp)  n_bits=t+b  bin_pt=b  preci_type=Single  exp_width=8  frac_width=24  explicit_period=off  period=1  equ=P=C  opselect=C  inp2=PCIN>>17  opr=+  inp1=P  carry=CIN  dbl_ovrd=off  block_type=constant
  x_imaginary : xbsIndex_r4/Slice  nbits=t+b  boolean_output=off  mode=Lower Bit Location + Width  bit1=0  base1=MSB of Input  bit0=0  base0=LSB of Input  dbl_ovrd=off  block_type=slice
  x_real : xbsIndex_r4/Slice  nbits=t+b  boolean_output=off  mode=Upper Bit Location + Width  bit1=0  base1=MSB of Input  bit0=0  base0=LSB of Input  dbl_ovrd=off  block_type=slice
  xWr : Outport
  xWi : Outport  Port=2
  wires:
  x_real/1 -> Reinterpret/1
  x_imaginary/1 -> Reinterpret1/1
  W_real/1 -> Mult1/2, Mult2/2
  x/1 -> x_real/1, x_imaginary/1
  Reinterpret/1 -> Mult/1, Mult2/1
  Reinterpret1/1 -> Mult1/1, Mult3/1
  W_imaginary/1 -> Mult/2, Mult3/2
  AddSub/1 -> xWi/1
  AddSub1/1 -> xWr/1
  Mult/1 -> AddSub/1
  Mult1/1 -> AddSub/2
  Mult3/1 -> AddSub1/2
  Mult2/1 -> AddSub1/1

== system dft_8_point/cplx mult50 ==
  x : Inport
  AddSub : xbsIndex_r4/AddSub  mode=Addition  use_carryin=off  use_carryout=off  en=off  latency=0  precision=User Defined  arith_type="Signed  (2's comp)"  n_bits=t+b+1  bin_pt=b  quantization=Truncate  overflow=Wrap  use_behavioral_HDL=off  hw_selection=Fabric  pipelined=off  dbl_ovrd=off  block_type=addsub
  AddSub1 : xbsIndex_r4/AddSub  mode=Subtraction  use_carryin=off  use_carryout=off  en=off  latency=0  precision=User Defined  arith_type="Signed  (2's comp)"  n_bits=t+b+1  bin_pt=b  quantization=Truncate  overflow=Wrap  use_behavioral_HDL=off  hw_selection=Fabric  pipelined=off  dbl_ovrd=off  block_type=addsub
  Mult{,1..3} (4 alike) : xbsIndex_r4/Mult  precision=User Defined  arith_type="Signed  (2's comp)"  n_bits=t+b  bin_pt=b  quantization=Truncate  overflow=Wrap  en=off  latency=0  use_behavioral_HDL=off  opt=Speed  use_embedded=on  optimum_pipeline=off  pipeline=on  dbl_ovrd=off  use_rpm=on  placement_style=Triangular  block_type=mult
  Reinterpret : xbsIndex_r4/Reinterpret  force_arith_type=on  arith_type="Signed  (2's comp)"  force_bin_pt=on  bin_pt=b  block_type=reinterpret
      settings: infoedit="Changes signal type without altering the binary representation.   You can changed the signal between signed and unsigned, and relocate the binary point.<br><br>Hardware notes: In hardware this block costs nothing.<br><br>Example:  Suppose the input is 6 bits wide, signed, with 2 fractional bits, and the output is forced to unsigned with 0 fractional bits.  Then an input of -2.0 (1110.00 in binary 2's complement) becomes an output of 56 (111000 in binary)."
  Reinterpret1 : xbsIndex_r4/Reinterpret  force_arith_type=on  arith_type="Signed  (2's comp)"  force_bin_pt=on  bin_pt=b  block_type=reinterpret
      settings: infoedit="Changes signal type without altering the binary representation.   You can changed the signal between signed and unsigned, and relocate the binary point.<br><br>Hardware notes: In hardware this block costs nothing.<br><br>Example:  Suppose the input is 6 bits wide, signed, with 2 fractional bits, and the output is forced to unsigned with 0 fractional bits.  Then an input of -2.0 (1110.00 in binary 2's complement) becomes an output of 56 (111000 in binary)."
  W_imaginary : xbsIndex_r4/Constant  const=imag(Wnk)  gui_display_data_type=Fixed-point  arith_type=Signed (2's comp)  n_bits=t+b  bin_pt=b  preci_type=Single  exp_width=8  frac_width=24  explicit_period=off  period=1  equ=P=C  opselect=C  inp2=PCIN>>17  opr=+  inp1=P  carry=CIN  dbl_ovrd=off  block_type=constant
  W_real : xbsIndex_r4/Constant  const=real(Wnk)  gui_display_data_type=Fixed-point  arith_type=Signed (2's comp)  n_bits=t+b  bin_pt=b  preci_type=Single  exp_width=8  frac_width=24  explicit_period=off  period=1  equ=P=C  opselect=C  inp2=PCIN>>17  opr=+  inp1=P  carry=CIN  dbl_ovrd=off  block_type=constant
  x_imaginary : xbsIndex_r4/Slice  nbits=t+b  boolean_output=off  mode=Lower Bit Location + Width  bit1=0  base1=MSB of Input  bit0=0  base0=LSB of Input  dbl_ovrd=off  block_type=slice
  x_real : xbsIndex_r4/Slice  nbits=t+b  boolean_output=off  mode=Upper Bit Location + Width  bit1=0  base1=MSB of Input  bit0=0  base0=LSB of Input  dbl_ovrd=off  block_type=slice
  xWr : Outport
  xWi : Outport  Port=2
  wires:
  x_real/1 -> Reinterpret/1
  x_imaginary/1 -> Reinterpret1/1
  W_real/1 -> Mult1/2, Mult2/2
  x/1 -> x_real/1, x_imaginary/1
  Reinterpret/1 -> Mult/1, Mult2/1
  Reinterpret1/1 -> Mult1/1, Mult3/1
  W_imaginary/1 -> Mult/2, Mult3/2
  AddSub/1 -> xWi/1
  AddSub1/1 -> xWr/1
  Mult/1 -> AddSub/1
  Mult1/1 -> AddSub/2
  Mult3/1 -> AddSub1/2
  Mult2/1 -> AddSub1/1

== system dft_8_point/cplx mult51 ==
  x : Inport
  AddSub : xbsIndex_r4/AddSub  mode=Addition  use_carryin=off  use_carryout=off  en=off  latency=0  precision=User Defined  arith_type="Signed  (2's comp)"  n_bits=t+b+1  bin_pt=b  quantization=Truncate  overflow=Wrap  use_behavioral_HDL=off  hw_selection=Fabric  pipelined=off  dbl_ovrd=off  block_type=addsub
  AddSub1 : xbsIndex_r4/AddSub  mode=Subtraction  use_carryin=off  use_carryout=off  en=off  latency=0  precision=User Defined  arith_type="Signed  (2's comp)"  n_bits=t+b+1  bin_pt=b  quantization=Truncate  overflow=Wrap  use_behavioral_HDL=off  hw_selection=Fabric  pipelined=off  dbl_ovrd=off  block_type=addsub
  Mult{,1..3} (4 alike) : xbsIndex_r4/Mult  precision=User Defined  arith_type="Signed  (2's comp)"  n_bits=t+b  bin_pt=b  quantization=Truncate  overflow=Wrap  en=off  latency=0  use_behavioral_HDL=off  opt=Speed  use_embedded=on  optimum_pipeline=off  pipeline=on  dbl_ovrd=off  use_rpm=on  placement_style=Triangular  block_type=mult
  Reinterpret : xbsIndex_r4/Reinterpret  force_arith_type=on  arith_type="Signed  (2's comp)"  force_bin_pt=on  bin_pt=b  block_type=reinterpret
      settings: infoedit="Changes signal type without altering the binary representation.   You can changed the signal between signed and unsigned, and relocate the binary point.<br><br>Hardware notes: In hardware this block costs nothing.<br><br>Example:  Suppose the input is 6 bits wide, signed, with 2 fractional bits, and the output is forced to unsigned with 0 fractional bits.  Then an input of -2.0 (1110.00 in binary 2's complement) becomes an output of 56 (111000 in binary)."
  Reinterpret1 : xbsIndex_r4/Reinterpret  force_arith_type=on  arith_type="Signed  (2's comp)"  force_bin_pt=on  bin_pt=b  block_type=reinterpret
      settings: infoedit="Changes signal type without altering the binary representation.   You can changed the signal between signed and unsigned, and relocate the binary point.<br><br>Hardware notes: In hardware this block costs nothing.<br><br>Example:  Suppose the input is 6 bits wide, signed, with 2 fractional bits, and the output is forced to unsigned with 0 fractional bits.  Then an input of -2.0 (1110.00 in binary 2's complement) becomes an output of 56 (111000 in binary)."
  W_imaginary : xbsIndex_r4/Constant  const=imag(Wnk)  gui_display_data_type=Fixed-point  arith_type=Signed (2's comp)  n_bits=t+b  bin_pt=b  preci_type=Single  exp_width=8  frac_width=24  explicit_period=off  period=1  equ=P=C  opselect=C  inp2=PCIN>>17  opr=+  inp1=P  carry=CIN  dbl_ovrd=off  block_type=constant
  W_real : xbsIndex_r4/Constant  const=real(Wnk)  gui_display_data_type=Fixed-point  arith_type=Signed (2's comp)  n_bits=t+b  bin_pt=b  preci_type=Single  exp_width=8  frac_width=24  explicit_period=off  period=1  equ=P=C  opselect=C  inp2=PCIN>>17  opr=+  inp1=P  carry=CIN  dbl_ovrd=off  block_type=constant
  x_imaginary : xbsIndex_r4/Slice  nbits=t+b  boolean_output=off  mode=Lower Bit Location + Width  bit1=0  base1=MSB of Input  bit0=0  base0=LSB of Input  dbl_ovrd=off  block_type=slice
  x_real : xbsIndex_r4/Slice  nbits=t+b  boolean_output=off  mode=Upper Bit Location + Width  bit1=0  base1=MSB of Input  bit0=0  base0=LSB of Input  dbl_ovrd=off  block_type=slice
  xWr : Outport
  xWi : Outport  Port=2
  wires:
  x_real/1 -> Reinterpret/1
  x_imaginary/1 -> Reinterpret1/1
  W_real/1 -> Mult1/2, Mult2/2
  x/1 -> x_real/1, x_imaginary/1
  Reinterpret/1 -> Mult/1, Mult2/1
  Reinterpret1/1 -> Mult1/1, Mult3/1
  W_imaginary/1 -> Mult/2, Mult3/2
  AddSub/1 -> xWi/1
  AddSub1/1 -> xWr/1
  Mult/1 -> AddSub/1
  Mult1/1 -> AddSub/2
  Mult3/1 -> AddSub1/2
  Mult2/1 -> AddSub1/1
